simulink model "simulate"  (R2023a)
settings: Solver=ode45  StartTime=0.0  StopTime=10.0  RelTol=1e-3  EnableMultiTasking=on
settings Model: Creator=nk  LastModifiedBy=zhs20
settings SolverCC: AlgebraicLoopSolver=TrustRegion
settings DataIOCC: LimitDataPoints=on  SaveFormat=Array  ReturnWorkspaceOutputs=off
settings OptimizationCC: LifeSpan=inf
settings DebuggingCC: SolverPrmCheckMsg=warning  UnconnectedInputMsg=warning  UnconnectedOutputMsg=warning  UnconnectedLineMsg=warning  SFUnexpectedBacktrackingDiag=warning  SFNoUnconditionalDefaultTransitionDiag=warning  SFExecutionAtInitializationDiag=none  ArithmeticOperatorsInVariantConditions=warning
settings HardwareCC: ProdBitPerPointer=32  ProdBitPerSizeT=32  ProdBitPerPtrDiffT=32  ProdLargestAtomicFloat=None  ProdIntDivRoundTo=Undefined  ProdEndianess=Unspecified  ProdWordSize=32  ProdHWDeviceType=32-bit Generic
settings ModelReferenceCC: PropagateSignalLabelsOutOfModel=off
settings SFSimCC: SimUseLocalCustomCode=off  CustomCodeUndefinedFunction=UseInterfaceOnly
settings RTWCC: RTWUseLocalCustomCode=off
settings CodeAppCC: StateflowObjectComments=on
settings GRTTargetCC: TargetLangStandard=C89/C90 (ANSI)
settings ConfigComp: CovMetricSettings=dw  CovSaveCumulativeToWorkspaceVar=on  CovSaveSingleToWorkspaceVar=on  CovExternalEMLEnable=off  CovSFcnEnable=off

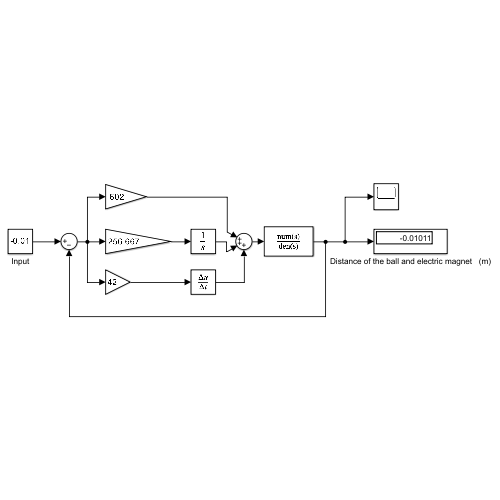
[thumbnail: Simulink's stored preview of the top-level diagram]
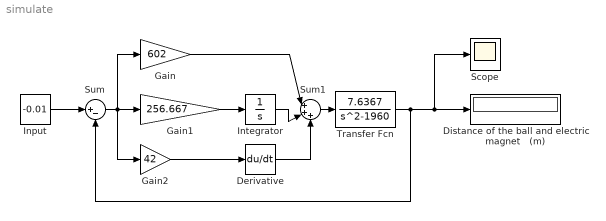
== system simulate ==
  Derivative : Derivative
  Distance of the ball and electric magnet   (m) : Display
      settings: Decimation=50
  Gain : Gain  Gain=602
  Gain1 : Gain  Gain=256.667
  Gain2 : Gain  Gain=42
  Input : Constant  Value=-0.01
  Integrator : Integrator
  Scope : Scope
  Sum : Sum  Inputs=|+-
  Sum1 : Sum  Inputs=|+++
  Transfer Fcn : TransferFcn  Numerator=[7.6367]  Denominator=[1 0 -1960]
  wires:
  Transfer Fcn/1 -> Scope/1, Distance of the ball and electric magnet   (m)/1, Sum/2
  Input/1 -> Sum/1
  Gain1/1 -> Integrator/1
  Sum/1 -> Gain1/1, Gain2/1, Gain/1
  Gain2/1 -> Derivative/1
  Sum1/1 -> Transfer Fcn/1
  Integrator/1 -> Sum1/2
  Derivative/1 -> Sum1/3
  Gain/1 -> Sum1/1
